simulink library "motohawk_control_primitives_lib"  (Simulink 7.5)
settings: Solver=ode45  SolverMode=SingleTasking  StartTime=0.0  StopTime=10.0  RelTol=1e-3
undefined symbols (not defined in the file): group, motohawk_vardec_config_group, motohawk_vardec_path, p, samp_time, SampleTime
libraries: MotoHawk_lib x103, motohawk_control_primitives_lib x29, simulink x11, AutoDoc_lib x4
(part 3 of 4)

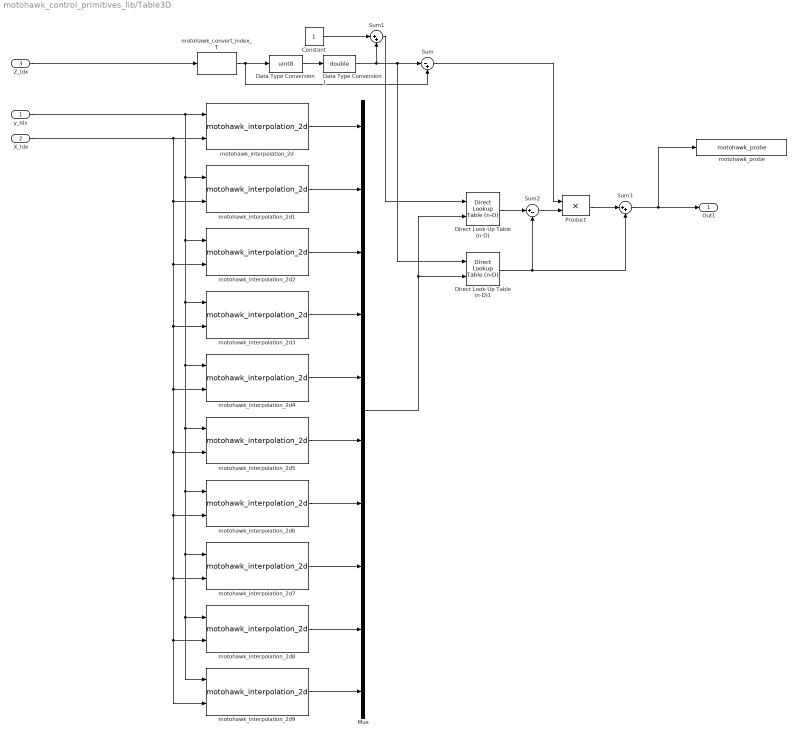
== system motohawk_control_primitives_lib/Table3D ==
  y_Idx : Inport  OutDataType=sfix(16)  OutScaling=2^0
  X_Idx : Inport  Port=2  OutDataType=sfix(16)  OutScaling=2^0
  Z_Idx : Inport  Port=3  OutDataType=sfix(16)  OutScaling=2^0
  Constant : Constant  OutDataType=sfix(16)  OutScaling=2^0
  Data Type Conversion : DataTypeConversion  OutDataTypeMode=uint8  OutDataType=sfix(16)  OutScaling=2^0  OutDataTypeStr=uint8  SaturateOnIntegerOverflow=on  RndMeth=Zero
  Data Type Conversion1 : DataTypeConversion  OutDataTypeMode=double  OutDataType=sfix(16)  OutScaling=2^0  OutDataTypeStr=double  SaturateOnIntegerOverflow=on  RndMeth=Zero
  Direct Look-Up Table (n-D) : simulink/Lookup Tables/Direct Lookup Table (n-D)  maskTabDims=1  explicitNumDims=1  outDims=Element  tabIsInput=on  mxTable=[4 5 6;16 19 20;10 18 23]  clipFlag=Warning
  Direct Look-Up Table (n-D)1 : simulink/Lookup Tables/Direct Lookup Table (n-D)  maskTabDims=1  explicitNumDims=1  outDims=Element  tabIsInput=on  mxTable=[4 5 6;16 19 20;10 18 23]  clipFlag=Warning
  Mux : Mux  Inputs=10
  Product : Product  OutDataType=sfix(16)  OutScaling=2^0  SaturateOnIntegerOverflow=on  OutDataTypeStr=Inherit: Same as first input
  Sum : Sum  Inputs=|-+  OutDataType=sfix(16)  OutScaling=2^0  SaturateOnIntegerOverflow=on
  Sum1 : Sum  Inputs=|++  OutDataType=sfix(16)  OutScaling=2^0  SaturateOnIntegerOverflow=on
  Sum2 : Sum  Inputs=|+-  OutDataType=sfix(16)  OutScaling=2^0  SaturateOnIntegerOverflow=on
  Sum3 : Sum  Inputs=|++  OutDataType=sfix(16)  OutScaling=2^0  SaturateOnIntegerOverflow=on
  motohawk_convert_index_T : MotoHawk_lib/Lookup Tables/motohawk_convert_index_T
  motohawk_interpolation_2d : MotoHawk_lib/Lookup Tables/motohawk_interpolation_2d  nam=[nam 'Z1']  table_data=table1data  show_more=on  data_type=Inherit from 'Table Data'  storage=NonAdaptive  read_level=1  write_level=1  ovr_cals=on  use_help=off  help=''  units=''  use_min_max=off  min_val=-inf  max_val=inf  use_precision=off  precision=''  gain=1  offset=0  exp=1  use_links=on  row_prelookup_block=rowprelookup  col_prelookup_block=colprelookup  output_name=''  use_mototune_group=on  mototune_group=grp
  motohawk_interpolation_2d1 : MotoHawk_lib/Lookup Tables/motohawk_interpolation_2d  nam=[nam 'Z2']  table_data=table2data  show_more=on  data_type=Inherit from 'Table Data'  storage=NonAdaptive  read_level=1  write_level=1  ovr_cals=on  use_help=off  help=''  units=''  use_min_max=off  min_val=-inf  max_val=inf  use_precision=off  precision=''  gain=1  offset=0  exp=1  use_links=on  row_prelookup_block=rowprelookup  col_prelookup_block=colprelookup  output_name=''  use_mototune_group=on  mototune_group=grp
  motohawk_interpolation_2d2 : MotoHawk_lib/Lookup Tables/motohawk_interpolation_2d  nam=[nam 'Z3']  table_data=table3data  show_more=on  data_type=Inherit from 'Table Data'  storage=NonAdaptive  read_level=1  write_level=1  ovr_cals=on  use_help=off  help=''  units=''  use_min_max=off  min_val=-inf  max_val=inf  use_precision=off  precision=''  gain=1  offset=0  exp=1  use_links=on  row_prelookup_block=rowprelookup  col_prelookup_block=colprelookup  output_name=''  use_mototune_group=on  mototune_group=grp
  motohawk_interpolation_2d3 : MotoHawk_lib/Lookup Tables/motohawk_interpolation_2d  nam=[nam 'Z4']  table_data=table4data  show_more=on  data_type=Inherit from 'Table Data'  storage=NonAdaptive  read_level=1  write_level=1  ovr_cals=on  use_help=off  help=''  units=''  use_min_max=off  min_val=-inf  max_val=inf  use_precision=off  precision=''  gain=1  offset=0  exp=1  use_links=on  row_prelookup_block=rowprelookup  col_prelookup_block=colprelookup  output_name=''  use_mototune_group=on  mototune_group=grp
  motohawk_interpolation_2d4 : MotoHawk_lib/Lookup Tables/motohawk_interpolation_2d  nam=[nam 'Z5']  table_data=table5data  show_more=on  data_type=Inherit from 'Table Data'  storage=NonAdaptive  read_level=1  write_level=1  ovr_cals=on  use_help=off  help=''  units=''  use_min_max=off  min_val=-inf  max_val=inf  use_precision=off  precision=''  gain=1  offset=0  exp=1  use_links=on  row_prelookup_block=rowprelookup  col_prelookup_block=colprelookup  output_name=''  use_mototune_group=on  mototune_group=grp
  motohawk_interpolation_2d5 : MotoHawk_lib/Lookup Tables/motohawk_interpolation_2d  nam=[nam 'Z6']  table_data=(table6data)  show_more=on  data_type=Inherit from 'Table Data'  storage=NonAdaptive  read_level=1  write_level=1  ovr_cals=on  use_help=off  help=''  units=''  use_min_max=off  min_val=-inf  max_val=inf  use_precision=off  precision=''  gain=1  offset=0  exp=1  use_links=on  row_prelookup_block=rowprelookup  col_prelookup_block=colprelookup  output_name=''  use_mototune_group=on  mototune_group=grp
  motohawk_interpolation_2d6 : MotoHawk_lib/Lookup Tables/motohawk_interpolation_2d  nam=[nam 'Z7']  table_data=(table7data)  show_more=on  data_type=Inherit from 'Table Data'  storage=NonAdaptive  read_level=1  write_level=1  ovr_cals=on  use_help=off  help=''  units=''  use_min_max=off  min_val=-inf  max_val=inf  use_precision=off  precision=''  gain=1  offset=0  exp=1  use_links=on  row_prelookup_block=rowprelookup  col_prelookup_block=colprelookup  output_name=''  use_mototune_group=on  mototune_group=grp
  motohawk_interpolation_2d7 : MotoHawk_lib/Lookup Tables/motohawk_interpolation_2d  nam=[nam 'Z8']  table_data=(table8data)  show_more=on  data_type=Inherit from 'Table Data'  storage=NonAdaptive  read_level=1  write_level=1  ovr_cals=on  use_help=off  help=''  units=''  use_min_max=off  min_val=-inf  max_val=inf  use_precision=off  precision=''  gain=1  offset=0  exp=1  use_links=on  row_prelookup_block=rowprelookup  col_prelookup_block=colprelookup  output_name=''  use_mototune_group=on  mototune_group=grp
  motohawk_interpolation_2d8 : MotoHawk_lib/Lookup Tables/motohawk_interpolation_2d  nam=[nam 'Z9']  table_data=(table9data)  show_more=on  data_type=Inherit from 'Table Data'  storage=NonAdaptive  read_level=1  write_level=1  ovr_cals=on  use_help=off  help=''  units=''  use_min_max=off  min_val=-inf  max_val=inf  use_precision=off  precision=''  gain=1  offset=0  exp=1  use_links=on  row_prelookup_block=rowprelookup  col_prelookup_block=colprelookup  output_name=''  use_mototune_group=on  mototune_group=grp
  motohawk_interpolation_2d9 : MotoHawk_lib/Lookup Tables/motohawk_interpolation_2d  nam=[nam 'Z10']  table_data=(table10data)  show_more=on  data_type=Inherit from 'Table Data'  storage=NonAdaptive  read_level=1  write_level=1  ovr_cals=on  use_help=off  help=''  units=''  use_min_max=off  min_val=-inf  max_val=inf  use_precision=off  precision=''  gain=1  offset=0  exp=1  use_links=on  row_prelookup_block=rowprelookup  col_prelookup_block=colprelookup  output_name=''  use_mototune_group=on  mototune_group=grp
  motohawk_probe : MotoHawk_lib/Calibration & Probing Blocks/motohawk_probe  nam=[nam]  show_more=on  name_source=Use Parameter  read_level=1  view_as=Number  enum_struct={'Disabled', 'Enabled'}  vector_style=Wide Row  use_help_units=off  help=''  units=''  use_header_enum=off  row_header_enum={}  col_header_enum={}  use_precision=off  precision=''  gain=1  offset=0  exp=1  use_mototune_group=on  mototune_group=grp
  Out1 : Outport  OutDataType=sfix(16)  OutScaling=2^0
  wires:
  Sum3/1 -> Out1/1, motohawk_probe/1
  Product/1 -> Sum3/1
  Direct Look-Up Table (n-D)1/1 -> Sum3/2, Sum2/2
  Direct Look-Up Table (n-D)/1 -> Sum2/1
  Sum1/1 -> Direct Look-Up Table (n-D)/1
  Constant/1 -> Sum1/1
  Data Type Conversion1/1 -> Direct Look-Up Table (n-D)1/1, Sum/1, Sum1/2
  Data Type Conversion/1 -> Data Type Conversion1/1
  motohawk_convert_index_T/1 -> Sum/2, Data Type Conversion/1
  motohawk_interpolation_2d3/1 -> Mux/4
  motohawk_interpolation_2d2/1 -> Mux/3
  motohawk_interpolation_2d1/1 -> Mux/2
  motohawk_interpolation_2d/1 -> Mux/1
  Z_Idx/1 -> motohawk_convert_index_T/1
  X_Idx/1 -> motohawk_interpolation_2d2/2, motohawk_interpolation_2d3/2, motohawk_interpolation_2d4/2, motohawk_interpolation_2d5/2, motohawk_interpolation_2d6/2, motohawk_interpolation_2d7/2, motohawk_interpolation_2d8/2, motohawk_interpolation_2d9/2, motohawk_interpolation_2d1/2, motohawk_interpolation_2d/2
  y_Idx/1 -> motohawk_interpolation_2d2/1, motohawk_interpolation_2d3/1, motohawk_interpolation_2d4/1, motohawk_interpolation_2d5/1, motohawk_interpolation_2d6/1, motohawk_interpolation_2d7/1, motohawk_interpolation_2d8/1, motohawk_interpolation_2d9/1, motohawk_interpolation_2d1/1, motohawk_interpolation_2d/1
  motohawk_interpolation_2d4/1 -> Mux/5
  motohawk_interpolation_2d5/1 -> Mux/6
  Sum/1 -> Product/1
  Sum2/1 -> Product/2
  motohawk_interpolation_2d6/1 -> Mux/7
  motohawk_interpolation_2d7/1 -> Mux/8
  motohawk_interpolation_2d8/1 -> Mux/9
  motohawk_interpolation_2d9/1 -> Mux/10
  Mux/1 -> Direct Look-Up Table (n-D)/2, Direct Look-Up Table (n-D)1/2

== system motohawk_control_primitives_lib/Time Since Enabled ==
  note: Output the time since enabled, by summing up 'dt'.
  note: If this block is in an enabled subsystem that
      | resets its states, then the count will reset as well.
      | Otherwise, the count will resume from where it left off.
      |
      | Note that when the Sample Time of the the 'dt' is non-positive,
      | the block will only output its Initial Value if the enabled subsystem
      | is set to reset its state.  This means that the count will immediately
      | 'catch up' if the enabled subsystem holds its states.
  Sum : Sum  Inputs=|++  OutDataType=sfix(16)  OutScaling=2^0  SaturateOnIntegerOverflow=on  InputSameDT=on
  Unit Delay : UnitDelay  SampleTime=-1
  motohawk_delta_time : MotoHawk_lib/Extra Development Blocks/motohawk_delta_time  samp_time=samp_time  init_val=0
  Time Since Enabled [sec] : Outport  OutDataType=sfix(16)  OutScaling=2^0
  wires:
  Unit Delay/1 -> Time Since Enabled [sec]/1, Sum/2
  Sum/1 -> Unit Delay/1
  motohawk_delta_time/1 -> Sum/1

== system motohawk_control_primitives_lib/Time Since Enabled (With Input) ==
  note: Output the time since enabled, by summing up 'dt'.
      | States are reset when re-enabled.
      | Output is reset to zero when disabled.
  Enable : EnablePort  StatesWhenEnabling=reset  ZeroCross=off
  Sum : Sum  Inputs=|++  OutDataType=sfix(16)  OutScaling=2^0  SaturateOnIntegerOverflow=on  InputSameDT=on
  Unit Delay : UnitDelay  SampleTime=-1
  motohawk_delta_time : MotoHawk_lib/Extra Development Blocks/motohawk_delta_time  samp_time=samp_time  init_val=0
  Time Since Enabled [sec] : Outport  OutDataType=sfix(16)  OutScaling=2^0  OutputWhenDisabled=reset  InitialOutput=init
  wires:
  motohawk_delta_time/1 -> Sum/1
  Sum/1 -> Unit Delay/1
  Unit Delay/1 -> Sum/2, Time Since Enabled [sec]/1

== system motohawk_control_primitives_lib/Time Since Enabled (With Input)1 ==
  Enable : Inport  OutDataType=sfix(16)  OutScaling=2^0
  Constant : Constant  Value=init  OutDataType=sfix(16)  OutScaling=2^0
  Saturation : Saturate  UpperLimit=upperlim  LowerLimit=0
  Sum : Sum  Inputs=++|  OutDataType=sfix(16)  OutScaling=2^0  SaturateOnIntegerOverflow=on  InputSameDT=on
  Switch : Switch  Threshold=1
  motohawk_data_def : MotoHawk_lib/Data Storage Blocks/motohawk_data_def  nam=nam  data=0  typ=double  struct_nam='MyStruct'  storage=Volatile  outputRef=off  use_vardec=off  window=Calibration  read_level=1  write_level=1  ovr_cals=on  view_as=Number  enum_struct={'Disabled', 'Enabled'}  vector_style=Wide Row  use_help_units=on  help=''  units=''  use_header_enum=off  row_header_enum=''  col_header_enum=''  use_min_max=off  min_val=-inf  max_val=inf  use_precision=off  precision=''  gain=1  offset=0  exp=1  use_mototune_group=off  mototune_group=motohawk_vardec_path(gcb)  eval_name=TimeSinceRun
  motohawk_data_read : MotoHawk_lib/Data Storage Blocks/motohawk_data_read  source=Lookup By Name  structure=Scalar  operation=Read scalar from location by index  sz_vec=4  sz_row=2  sz_col=3  typ=double  nam=nam  checkNull=on  struct_inst_name='Struct1'
  motohawk_data_write : MotoHawk_lib/Data Storage Blocks/motohawk_data_write  source=Lookup By Name  structure=Scalar  operation=Write scalar into location by index  sz_vec=-1  sz_row=3  sz_col=2  typ=double  nam=nam  checkNull=on  write_read_only=off  struct_inst_name='Struct1'
  motohawk_delta_time : MotoHawk_lib/Extra Development Blocks/motohawk_delta_time  samp_time=samp_time  init_val=.005
  Time : Outport  OutDataType=sfix(16)  OutScaling=2^0  OutputWhenDisabled=reset  InitialOutput=init
  wires:
  motohawk_delta_time/1 -> Sum/1
  motohawk_data_read/1 -> Sum/2
  Switch/1 -> Time/1, Saturation/1
  Enable/1 -> Switch/2
  Sum/1 -> Switch/1
  Constant/1 -> Switch/3
  Saturation/1 -> motohawk_data_write/1

== system motohawk_control_primitives_lib/Triggered Counter Falling ==
  note: Triggered Counter
  Reset : Inport  OutDataType=sfix(16)  OutScaling=2^0
  Increment : Inport  Port=2  OutDataType=sfix(16)  OutScaling=2^0
  Trigger : TriggerPort  TriggerType=falling
  Constant : Constant  Value=0  OutDataType=sfix(16)  OutScaling=2^0
  Sum : Sum  OutDataType=sfix(16)  OutScaling=2^0  SaturateOnIntegerOverflow=on  InputSameDT=on  OutDataTypeStr=Inherit: Same as first input
  Switch : Switch  Threshold=0.5  SaturateOnIntegerOverflow=on  InputSameDT=on
  Unit Delay1 : UnitDelay  SampleTime=-1
  Counter : Outport  OutDataType=sfix(16)  OutScaling=2^0
  wires:
  Unit Delay1/1 -> Sum/2
  Increment/1 -> Sum/1
  Reset/1 -> Switch/2
  Switch/1 -> Unit Delay1/1, Counter/1
  Constant/1 -> Switch/1
  Sum/1 -> Switch/3

== system motohawk_control_primitives_lib/Triggered Counter Rising ==
  note: Triggered Counter
  Reset : Inport  OutDataType=sfix(16)  OutScaling=2^0
  Increment : Inport  Port=2  OutDataType=sfix(16)  OutScaling=2^0
  Trigger : TriggerPort
  Constant : Constant  Value=0  OutDataType=sfix(16)  OutScaling=2^0
  Sum : Sum  OutDataType=sfix(16)  OutScaling=2^0  SaturateOnIntegerOverflow=on  InputSameDT=on  OutDataTypeStr=Inherit: Same as first input
  Switch : Switch  Threshold=0.5  SaturateOnIntegerOverflow=on  InputSameDT=on
  Unit Delay1 : UnitDelay  SampleTime=-1
  Counter : Outport  OutDataType=sfix(16)  OutScaling=2^0
  wires:
  Switch/1 -> Counter/1, Unit Delay1/1
  Reset/1 -> Switch/2
  Constant/1 -> Switch/1
  Sum/1 -> Switch/3
  Increment/1 -> Sum/1
  Unit Delay1/1 -> Sum/2

== system motohawk_control_primitives_lib/Universal PD ==
  note: Universal PD Controller
  Actual : Inport  OutDataType=sfix(16)  OutScaling=2^0
  SetPt : Inport  Port=2  OutDataType=sfix(16)  OutScaling=2^0
  k_Err : Inport  Port=3  OutDataType=sfix(16)  OutScaling=2^0
  k_P : Inport  Port=4  OutDataType=sfix(16)  OutScaling=2^0
  k_D : Inport  Port=5  OutDataType=sfix(16)  OutScaling=2^0
  Data Type Conversion : DataTypeConversion  OutDataType=sfix(16)  OutScaling=2^0  SaturateOnIntegerOverflow=on  RndMeth=Zero
  Derivitive : motohawk_control_primitives_lib/Derivitive  samp_time=samp_time
  Model Info : simulink/Model-Wide Utilities/Model Info  InitialBlockCM=None  BlockCM=None  Frame=on  DisplayStringWithTags=|  HorizontalTextAlignment=Center  LeftAlignmentValue=0.5  SourceBlockDiagram=motohawk_control_primitives_lib  TagMaxNumber=20
      | Model Info:
      | Author: %<Creator>
      | %<Created>
      | %<ModifiedDate>
      | Version: %<ModelVersion>
      | MotoTron Confidential
      | and Propietary
  Product : Product  OutDataType=sfix(16)  OutScaling=2^0  InputSameDT=on  OutDataTypeStr=Inherit: Same as first input
  Product2 : Product  OutDataType=sfix(16)  OutScaling=2^0  InputSameDT=on  OutDataTypeStr=Inherit: Same as first input
  Product4 : Product  OutDataType=sfix(16)  OutScaling=2^0  InputSameDT=on  OutDataTypeStr=Inherit: Same as first input
  Sum : Sum  OutDataType=sfix(16)  OutScaling=2^0  SaturateOnIntegerOverflow=on  InputSameDT=on  OutDataTypeStr=Inherit: Same as first input
  Sum1 : Sum  Inputs=|-+  OutDataType=sfix(16)  OutScaling=2^0
  Out : Outport  OutDataType=sfix(16)  OutScaling=2^0
  Err : Outport  Port=2  OutDataType=sfix(16)  OutScaling=2^0
  P_term : Outport  Port=3  OutDataType=sfix(16)  OutScaling=2^0
  D_term : Outport  Port=4  OutDataType=sfix(16)  OutScaling=2^0
  wires:
  Product4/1 -> Product2/1, Product/1
  Sum/1 -> Out/1
  Derivitive/1 -> Sum/2, D_term/1
  Product/1 -> Sum/1, P_term/1
  Product2/1 -> Derivitive/1
  k_D/1 -> Product2/2
  k_P/1 -> Product/2
  Actual/1 -> Sum1/1
  SetPt/1 -> Sum1/2
  Sum1/1 -> Data Type Conversion/1
  k_Err/1 -> Product4/2
  Data Type Conversion/1 -> Product4/1, Err/1

== system motohawk_control_primitives_lib/Universal PD (Tunable & Scheduled) ==
  note: Universal PD Feedback Control
      | With Calibratable Parameters,
      | Gain Schedules, and Observable States
  Actual : Inport  OutDataType=sfix(16)  OutScaling=2^0
  SetPoint : Inport  Port=2  OutDataType=sfix(16)  OutScaling=2^0
  Product1 : Product  OutDataType=sfix(16)  OutScaling=2^0  SaturateOnIntegerOverflow=on  InputSameDT=on  OutDataTypeStr=Inherit: Same as first input
  Product2 : Product  OutDataType=sfix(16)  OutScaling=2^0  SaturateOnIntegerOverflow=on  InputSameDT=on  OutDataTypeStr=Inherit: Same as first input
  Saturation (Tunable) : motohawk_control_primitives_lib/Saturation (Tunable)  prefix=prefix  units=units  grp=motohawk_vardec_config_group(grp)
  Sum : Sum  Inputs=++|  OutDataType=sfix(16)  OutScaling=2^0  InputSameDT=on
  Universal PD : motohawk_control_primitives_lib/Universal PD  Description=|  samp_time=SampleTime
      | /* Name: ErrorGain Unit:mult ClassID:VAR StorageID:FLASH Access:RW4+RW3+NA2+NA1 TypeID:UINT4                   
      |    Gain:0.000000001 Min:0.000000000 Max:4.000000000 Format:10.9 UpdateID:REMOTE Help:"This gain is applied to "
      |    "the error term before it is used to calculate the P, I and D terms." VardecSig:6C */                       
      |                                                                                                                
      | /* Name: ITermLowerLim Unit:0 ClassID:VAR StorageID:FLASH Access:RW4+RW3+NA2+NA1 TypeID:SINT2 Gain:0.1         
      |    Min:-3276.8 Max:3276.7 Format:5.1 UpdateID:REMOTE Help:"Lower limit on the I-term value." VardecSig:6C */   
      |                                                                                                                
      | /* Name: ITermUpperLim ClassID:VAR StorageID:FLASH Access:RW4+RW3+NA2+NA1 TypeID:SINT2 Gain:0.1 Min:-3276.8    
      |    Max:3276.7 Format:5.1 UpdateID:REMOTE Help:"Upper limit on I-term value." VardecSig:6C */                   
      |                                                                                                                
      | /* Name: PIDOutLowerLim ClassID:VAR StorageID:FLASH Access:RW4+RW3+NA2+NA1 TypeID:SINT2 Gain:0.1               
      |    Min:-3276.8 Max:3276.7 Format:5.1 UpdateID:REMOTE Help:"Lower limit on PID output." VardecSig:6C */         
      |                                                                                                                
      | /* Name: PIDOutUpperLim ClassID:VAR StorageID:FLASH Access:RW4+RW3+NA2+NA1 TypeID:SINT2 Gain:0.1               
      |    Min:-3276.8 Max:3276.7 Format:3.1 UpdateID:REMOTE Help:"Upper limit on PID output." VardecSig:6C */
  motohawk_calibration : MotoHawk_lib/Calibration & Probing Blocks/motohawk_calibration  nam=[prefix 'PGain']  val=1  storage=Calibration  show_more=on  name_source=Use Parameter  data_type=Inherit from 'Default Value'  read_level=1  write_level=1  ovr_cals=on  view_as=Number  enum_struct={'Disabled', 'Enabled'}  vector_style=Wide Row  use_help_units=on  help='PID Proportional Gain'  units='mult'  use_header_enum=off  row_header_enum={}  col_header_enum={}  use_min_max=off  min_val=-inf  max_val=inf  use_precision=off  precision=''  gain=1  offset=0  exp=1  use_mototune_group=on  mototune_group=motohawk_vardec_config_group(grp)
  motohawk_calibration1 : MotoHawk_lib/Calibration & Probing Blocks/motohawk_calibration  nam=[prefix 'DGain']  val=1  storage=Calibration  show_more=on  name_source=Use Parameter  data_type=Inherit from 'Default Value'  read_level=1  write_level=1  ovr_cals=on  view_as=Number  enum_struct={'Disabled', 'Enabled'}  vector_style=Wide Row  use_help_units=on  help='PID Derivative Gain'  units='mult'  use_header_enum=off  row_header_enum={}  col_header_enum={}  use_min_max=off  min_val=-inf  max_val=inf  use_precision=off  precision=''  gain=1  offset=0  exp=1  use_mototune_group=on  mototune_group=motohawk_vardec_config_group(grp)
  motohawk_calibration5 : MotoHawk_lib/Calibration & Probing Blocks/motohawk_calibration  nam=[prefix 'DCOffset']  val=0  storage=Calibration  show_more=on  name_source=Use Parameter  data_type=Inherit from 'Default Value'  read_level=1  write_level=1  ovr_cals=on  view_as=Number  enum_struct={'Disabled', 'Enabled'}  vector_style=Wide Row  use_help_units=on  help='PID Output DC Offset'  units=units  use_header_enum=off  row_header_enum={}  col_header_enum={}  use_min_max=off  min_val=-inf  max_val=inf  use_precision=off  precision=''  gain=1  offset=0  exp=1  use_mototune_group=on  mototune_group=motohawk_vardec_config_group(grp)
  motohawk_calibration6 : MotoHawk_lib/Calibration & Probing Blocks/motohawk_calibration  nam=[prefix 'ErrorGain']  val=1  storage=Calibration  show_more=on  name_source=Use Parameter  data_type=Inherit from 'Default Value'  read_level=1  write_level=1  ovr_cals=on  view_as=Number  enum_struct={'Disabled', 'Enabled'}  vector_style=Wide Row  use_help_units=on  help='PID Error Gain'  units='mult'  use_header_enum=off  row_header_enum={}  col_header_enum={}  use_min_max=off  min_val=-inf  max_val=inf  use_precision=off  precision=''  gain=1  offset=0  exp=1  use_mototune_group=on  mototune_group=motohawk_vardec_config_group(grp)
  motohawk_interpolation_1d : MotoHawk_lib/Lookup Tables/motohawk_interpolation_1d  nam=[prefix 'PMult']  table_data=ones(1,tblsize)  show_more=on  data_type=Inherit from 'Table Data'  storage=NonAdaptive  read_level=1  write_level=1  ovr_cals=on  use_help=on  help='Proportional term gain schedule'  units='mult'  use_min_max=off  min_val=-inf  max_val=inf  use_precision=off  precision=''  gain=1  offset=0  exp=1  use_links=off  prelookup_block=''  output_name=''  use_mototune_group=on  mototune_group=grp
  motohawk_interpolation_1d1 : MotoHawk_lib/Lookup Tables/motohawk_interpolation_1d  nam=[prefix 'DMult']  table_data=ones(1,tblsize)  show_more=on  data_type=Inherit from 'Table Data'  storage=NonAdaptive  read_level=1  write_level=1  ovr_cals=on  use_help=on  help='Derivative term gain schedule'  units='mult'  use_min_max=off  min_val=-inf  max_val=inf  use_precision=off  precision=''  gain=1  offset=0  exp=1  use_links=off  prelookup_block=''  output_name=''  use_mototune_group=on  mototune_group=grp
  motohawk_prelookup : MotoHawk_lib/Lookup Tables/motohawk_prelookup  nam=[prefix 'Error']  breakpoint_data=ones(1,tblsize)  show_more=on  data_type=Inherit from 'Table Data'  storage=Constant  read_level=1  write_level=1  ovr_cals=on  use_help=on  help='Error gain schedule ordinates'  units=units  use_min_max=off  min_val=-inf  max_val=inf  use_precision=off  precision=''  gain=1  offset=0  exp=1  use_links=on  input_name=[prefix 'Error']  use_mototune_group=on  mototune_group=grp
  motohawk_probe : MotoHawk_lib/Calibration & Probing Blocks/motohawk_probe  nam=[prefix 'Out']  show_more=on  name_source=Use Parameter  read_level=1  view_as=Number  enum_struct={'Disabled', 'Enabled'}  vector_style=Wide Row  use_help_units=on  help='PID Final Output'  units=units  use_header_enum=off  row_header_enum={}  col_header_enum={}  use_precision=off  precision=''  gain=1  offset=0  exp=1  use_mototune_group=on  mototune_group=grp
  motohawk_probe1 : MotoHawk_lib/Calibration & Probing Blocks/motohawk_probe  nam=[prefix 'PTerm']  show_more=on  name_source=Use Parameter  read_level=1  view_as=Number  enum_struct={'Disabled', 'Enabled'}  vector_style=Wide Row  use_help_units=on  help='PID Proportional Term'  units=units  use_header_enum=off  row_header_enum={}  col_header_enum={}  use_precision=off  precision=''  gain=1  offset=0  exp=1  use_mototune_group=on  mototune_group=grp
  motohawk_probe3 : MotoHawk_lib/Calibration & Probing Blocks/motohawk_probe  nam=[prefix 'DTerm']  show_more=on  name_source=Use Parameter  read_level=1  view_as=Number  enum_struct={'Disabled', 'Enabled'}  vector_style=Wide Row  use_help_units=on  help='PID Derivative Term'  units=units  use_header_enum=off  row_header_enum={}  col_header_enum={}  use_precision=off  precision=''  gain=1  offset=0  exp=1  use_mototune_group=on  mototune_group=grp
  motohawk_probe4 : MotoHawk_lib/Calibration & Probing Blocks/motohawk_probe  nam=[prefix 'Error']  show_more=on  name_source=Use Parameter  read_level=1  view_as=Number  enum_struct={'Disabled', 'Enabled'}  vector_style=Wide Row  use_help_units=on  help='PID Error Term'  units=units  use_header_enum=off  row_header_enum={}  col_header_enum={}  use_precision=off  precision=''  gain=1  offset=0  exp=1  use_mototune_group=on  mototune_group=grp
  Out : Outport  OutDataType=sfix(16)  OutScaling=2^0
  wires:
  motohawk_prelookup/1 -> motohawk_interpolation_1d1/1, motohawk_interpolation_1d/1
  SetPoint/1 -> Universal PD/2
  Actual/1 -> Universal PD/1
  Saturation (Tunable)/1 -> motohawk_probe/1, Out/1
  Universal PD/2 -> motohawk_prelookup/1, motohawk_probe4/1
  Universal PD/4 -> motohawk_probe3/1
  Universal PD/1 -> Sum/2
  Universal PD/3 -> motohawk_probe1/1
  Sum/1 -> Saturation (Tunable)/1
  motohawk_calibration5/1 -> Sum/1
  motohawk_calibration6/1 -> Universal PD/3
  Product2/1 -> Universal PD/4
  motohawk_calibration/1 -> Product2/1
  Product1/1 -> Universal PD/5
  motohawk_calibration1/1 -> Product1/1
  motohawk_interpolation_1d/1 -> Product2/2
  motohawk_interpolation_1d1/1 -> Product1/2

== system motohawk_control_primitives_lib/Universal PD (Tunable) ==
  note: Universal PD Feedback Control
      | With Calibratable Parameters and Observable States
  Actual : Inport  OutDataType=sfix(16)  OutScaling=2^0
  SetPoint : Inport  Port=2  OutDataType=sfix(16)  OutScaling=2^0
  Saturation (Tunable) : motohawk_control_primitives_lib/Saturation (Tunable)  prefix=prefix  units=units  grp=grp
  Sum : Sum  Inputs=++|  OutDataType=sfix(16)  OutScaling=2^0  InputSameDT=on
  Universal PD : motohawk_control_primitives_lib/Universal PD  Description=|  samp_time=SampleTime
      | /* Name: ErrorGain Unit:mult ClassID:VAR StorageID:FLASH Access:RW4+RW3+NA2+NA1 TypeID:UINT4                   
      |    Gain:0.000000001 Min:0.000000000 Max:4.000000000 Format:10.9 UpdateID:REMOTE Help:"This gain is applied to "
      |    "the error term before it is used to calculate the P, I and D terms." VardecSig:6C */                       
      |                                                                                                                
      | /* Name: ITermLowerLim Unit:0 ClassID:VAR StorageID:FLASH Access:RW4+RW3+NA2+NA1 TypeID:SINT2 Gain:0.1         
      |    Min:-3276.8 Max:3276.7 Format:5.1 UpdateID:REMOTE Help:"Lower limit on the I-term value." VardecSig:6C */   
      |                                                                                                                
      | /* Name: ITermUpperLim ClassID:VAR StorageID:FLASH Access:RW4+RW3+NA2+NA1 TypeID:SINT2 Gain:0.1 Min:-3276.8    
      |    Max:3276.7 Format:5.1 UpdateID:REMOTE Help:"Upper limit on I-term value." VardecSig:6C */                   
      |                                                                                                                
      | /* Name: PIDOutLowerLim ClassID:VAR StorageID:FLASH Access:RW4+RW3+NA2+NA1 TypeID:SINT2 Gain:0.1               
      |    Min:-3276.8 Max:3276.7 Format:5.1 UpdateID:REMOTE Help:"Lower limit on PID output." VardecSig:6C */         
      |                                                                                                                
      | /* Name: PIDOutUpperLim ClassID:VAR StorageID:FLASH Access:RW4+RW3+NA2+NA1 TypeID:SINT2 Gain:0.1               
      |    Min:-3276.8 Max:3276.7 Format:3.1 UpdateID:REMOTE Help:"Upper limit on PID output." VardecSig:6C */
  motohawk_calibration : MotoHawk_lib/Calibration & Probing Blocks/motohawk_calibration  nam=[prefix 'PGain']  val=1  storage=Calibration  show_more=on  name_source=Use Parameter  data_type=Inherit from 'Default Value'  read_level=1  write_level=1  ovr_cals=on  view_as=Number  enum_struct={'Disabled', 'Enabled'}  vector_style=Wide Row  use_help_units=on  help='PID Proportional Gain'  units='mult'  use_header_enum=off  row_header_enum={}  col_header_enum={}  use_min_max=off  min_val=-inf  max_val=inf  use_precision=off  precision=''  gain=1  offset=0  exp=1  use_mototune_group=on  mototune_group=grp
  motohawk_calibration1 : MotoHawk_lib/Calibration & Probing Blocks/motohawk_calibration  nam=[prefix 'DGain']  val=1  storage=Calibration  show_more=on  name_source=Use Parameter  data_type=Inherit from 'Default Value'  read_level=1  write_level=1  ovr_cals=on  view_as=Number  enum_struct={'Disabled', 'Enabled'}  vector_style=Wide Row  use_help_units=on  help='PID Derivative Gain'  units='mult'  use_header_enum=off  row_header_enum={}  col_header_enum={}  use_min_max=off  min_val=-inf  max_val=inf  use_precision=off  precision=''  gain=1  offset=0  exp=1  use_mototune_group=on  mototune_group=grp
  motohawk_calibration5 : MotoHawk_lib/Calibration & Probing Blocks/motohawk_calibration  nam=[prefix 'DCOffset']  val=0  storage=Calibration  show_more=on  name_source=Use Parameter  data_type=Inherit from 'Default Value'  read_level=1  write_level=1  ovr_cals=on  view_as=Number  enum_struct={'Disabled', 'Enabled'}  vector_style=Wide Row  use_help_units=on  help='PID Output DC Offset'  units=units  use_header_enum=off  row_header_enum={}  col_header_enum={}  use_min_max=off  min_val=-inf  max_val=inf  use_precision=off  precision=''  gain=1  offset=0  exp=1  use_mototune_group=on  mototune_group=grp
  motohawk_calibration6 : MotoHawk_lib/Calibration & Probing Blocks/motohawk_calibration  nam=[prefix 'ErrorGain']  val=1  storage=Calibration  show_more=on  name_source=Use Parameter  data_type=Inherit from 'Default Value'  read_level=1  write_level=1  ovr_cals=on  view_as=Number  enum_struct={'Disabled', 'Enabled'}  vector_style=Wide Row  use_help_units=on  help='PID Error Gain'  units='mult'  use_header_enum=off  row_header_enum={}  col_header_enum={}  use_min_max=off  min_val=-inf  max_val=inf  use_precision=off  precision=''  gain=1  offset=0  exp=1  use_mototune_group=on  mototune_group=grp
  motohawk_probe : MotoHawk_lib/Calibration & Probing Blocks/motohawk_probe  nam=[prefix 'Out']  show_more=on  name_source=Use Parameter  read_level=1  view_as=Number  enum_struct={'Disabled', 'Enabled'}  vector_style=Wide Row  use_help_units=on  help='PID Final Output'  units=units  use_header_enum=off  row_header_enum={}  col_header_enum={}  use_precision=off  precision=''  gain=1  offset=0  exp=1  use_mototune_group=on  mototune_group=grp
  motohawk_probe1 : MotoHawk_lib/Calibration & Probing Blocks/motohawk_probe  nam=[prefix 'PTerm']  show_more=on  name_source=Use Parameter  read_level=1  view_as=Number  enum_struct={'Disabled', 'Enabled'}  vector_style=Wide Row  use_help_units=on  help='PID Proportional Term'  units=units  use_header_enum=off  row_header_enum={}  col_header_enum={}  use_precision=off  precision=''  gain=1  offset=0  exp=1  use_mototune_group=on  mototune_group=grp
  motohawk_probe3 : MotoHawk_lib/Calibration & Probing Blocks/motohawk_probe  nam=[prefix 'DTerm']  show_more=on  name_source=Use Parameter  read_level=1  view_as=Number  enum_struct={'Disabled', 'Enabled'}  vector_style=Wide Row  use_help_units=on  help='PID Derivative Term'  units=units  use_header_enum=off  row_header_enum={}  col_header_enum={}  use_precision=off  precision=''  gain=1  offset=0  exp=1  use_mototune_group=on  mototune_group=grp
  motohawk_probe4 : MotoHawk_lib/Calibration & Probing Blocks/motohawk_probe  nam=[prefix 'Error']  show_more=on  name_source=Use Parameter  read_level=1  view_as=Number  enum_struct={'Disabled', 'Enabled'}  vector_style=Wide Row  use_help_units=on  help='PID Error Term'  units=units  use_header_enum=off  row_header_enum={}  col_header_enum={}  use_precision=off  precision=''  gain=1  offset=0  exp=1  use_mototune_group=on  mototune_group=grp
  Out : Outport  OutDataType=sfix(16)  OutScaling=2^0
  wires:
  motohawk_calibration5/1 -> Sum/1
  Sum/1 -> Saturation (Tunable)/1
  Universal PD/3 -> motohawk_probe1/1
  Universal PD/1 -> Sum/2
  Universal PD/4 -> motohawk_probe3/1
  Universal PD/2 -> motohawk_probe4/1
  Saturation (Tunable)/1 -> Out/1, motohawk_probe/1
  motohawk_calibration6/1 -> Universal PD/3
  motohawk_calibration/1 -> Universal PD/4
  motohawk_calibration1/1 -> Universal PD/5
  Actual/1 -> Universal PD/1
  SetPoint/1 -> Universal PD/2

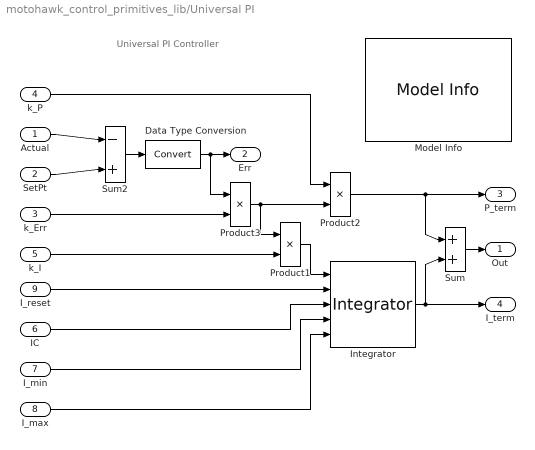
== system motohawk_control_primitives_lib/Universal PI ==
  note: Universal PI Controller
  Actual : Inport  OutDataType=sfix(16)  OutScaling=2^0
  SetPt : Inport  Port=2  OutDataType=sfix(16)  OutScaling=2^0
  k_Err : Inport  Port=3  OutDataType=sfix(16)  OutScaling=2^0
  k_P : Inport  Port=4  OutDataType=sfix(16)  OutScaling=2^0
  k_I : Inport  Port=5  OutDataType=sfix(16)  OutScaling=2^0
  IC : Inport  Port=6  OutDataType=sfix(16)  OutScaling=2^0
  I_min : Inport  Port=7  OutDataType=sfix(16)  OutScaling=2^0
  I_max : Inport  Port=8  OutDataType=sfix(16)  OutScaling=2^0
  I_reset : Inport  Port=9  OutDataType=sfix(16)  OutScaling=2^0
  Data Type Conversion : DataTypeConversion  OutDataType=sfix(16)  OutScaling=2^0  SaturateOnIntegerOverflow=on  RndMeth=Zero
  Integrator : motohawk_control_primitives_lib/Integrator  samp_time=samp_time
  Model Info : simulink/Model-Wide Utilities/Model Info  InitialBlockCM=None  BlockCM=None  Frame=on  DisplayStringWithTags=|  HorizontalTextAlignment=Center  LeftAlignmentValue=0.5  SourceBlockDiagram=motohawk_control_primitives_lib  TagMaxNumber=20
      | Model Info:
      | Author: Poorman
      | %<Created>
      | %<ModifiedDate>
      | Version: %<ModelVersion>
      | MotoTron Confidential
      | and Propietary
  Product1 : Product  OutDataType=sfix(16)  OutScaling=2^0  InputSameDT=on  OutDataTypeStr=Inherit: Same as first input
  Product2 : Product  OutDataType=sfix(16)  OutScaling=2^0  InputSameDT=on  OutDataTypeStr=Inherit: Same as first input
  Product3 : Product  OutDataType=sfix(16)  OutScaling=2^0  InputSameDT=on  OutDataTypeStr=Inherit: Same as first input
  Sum : Sum  Inputs=+|+  OutDataType=sfix(16)  OutScaling=2^0  SaturateOnIntegerOverflow=on  InputSameDT=on  OutDataTypeStr=Inherit: Same as first input
  Sum2 : Sum  Inputs=-|+  OutDataType=sfix(16)  OutScaling=2^0  SaturateOnIntegerOverflow=on  InputSameDT=on  OutDataTypeStr=Inherit: Same as first input
  Out : Outport  OutDataType=sfix(16)  OutScaling=2^0
  Err : Outport  Port=2  OutDataType=sfix(16)  OutScaling=2^0
  P_term : Outport  Port=3  OutDataType=sfix(16)  OutScaling=2^0
  I_term : Outport  Port=4  OutDataType=sfix(16)  OutScaling=2^0
  wires:
  I_max/1 -> Integrator/5
  I_min/1 -> Integrator/4
  Data Type Conversion/1 -> Err/1, Product3/1
  k_Err/1 -> Product3/2
  I_reset/1 -> Integrator/2
  SetPt/1 -> Sum2/2
  Actual/1 -> Sum2/1
  k_P/1 -> Product2/1
  k_I/1 -> Product1/2
  Product1/1 -> Integrator/1
  Product2/1 -> P_term/1, Sum/1
  Integrator/1 -> I_term/1, Sum/2
  Sum/1 -> Out/1
  IC/1 -> Integrator/3
  Product3/1 -> Product2/2, Product1/1
  Sum2/1 -> Data Type Conversion/1

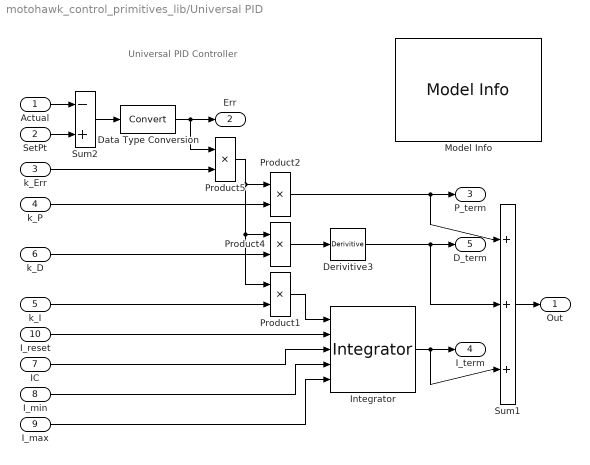
== system motohawk_control_primitives_lib/Universal PID ==
  note: Universal PID Controller
  Actual : Inport  OutDataType=sfix(16)  OutScaling=2^0
  SetPt : Inport  Port=2  OutDataType=sfix(16)  OutScaling=2^0
  k_Err : Inport  Port=3  OutDataType=sfix(16)  OutScaling=2^0
  k_P : Inport  Port=4  OutDataType=sfix(16)  OutScaling=2^0
  k_I : Inport  Port=5  OutDataType=sfix(16)  OutScaling=2^0
  k_D : Inport  Port=6  OutDataType=sfix(16)  OutScaling=2^0
  IC : Inport  Port=7  OutDataType=sfix(16)  OutScaling=2^0
  I_min : Inport  Port=8  OutDataType=sfix(16)  OutScaling=2^0
  I_max : Inport  Port=9  OutDataType=sfix(16)  OutScaling=2^0
  I_reset : Inport  Port=10  OutDataType=sfix(16)  OutScaling=2^0
  Data Type Conversion : DataTypeConversion  OutDataType=sfix(16)  OutScaling=2^0  SaturateOnIntegerOverflow=on  RndMeth=Zero
  Derivitive3 : motohawk_control_primitives_lib/Derivitive  samp_time=samp_time
  Integrator : motohawk_control_primitives_lib/Integrator  samp_time=samp_time
  Model Info : simulink/Model-Wide Utilities/Model Info  InitialBlockCM=None  BlockCM=None  Frame=on  DisplayStringWithTags=|  HorizontalTextAlignment=Center  LeftAlignmentValue=0.5  SourceBlockDiagram=motohawk_control_primitives_lib  TagMaxNumber=20
      | Model Info:
      | Author: Suhre, Poorman
      | %<Created>
      | %<ModifiedDate>
      | Version: %<ModelVersion>
      | MotoTron Confidential
      | and Propietary
  Product{1..2,4..5} (4 alike) : Product  OutDataType=sfix(16)  OutScaling=2^0  InputSameDT=on  OutDataTypeStr=Inherit: Same as first input
  Sum1 : Sum  Inputs=+|+|+  OutDataType=sfix(16)  OutScaling=2^0  SaturateOnIntegerOverflow=on  InputSameDT=on  OutDataTypeStr=Inherit: Same as first input
  Sum2 : Sum  Inputs=-+  OutDataType=sfix(16)  OutScaling=2^0  SaturateOnIntegerOverflow=on  InputSameDT=on  OutDataTypeStr=Inherit: Same as first input
  Out : Outport  OutDataType=sfix(16)  OutScaling=2^0
  Err : Outport  Port=2  OutDataType=sfix(16)  OutScaling=2^0
  P_term : Outport  Port=3  OutDataType=sfix(16)  OutScaling=2^0
  I_term : Outport  Port=4  OutDataType=sfix(16)  OutScaling=2^0
  D_term : Outport  Port=5  OutDataType=sfix(16)  OutScaling=2^0
  wires:
  I_max/1 -> Integrator/5
  I_min/1 -> Integrator/4
  Data Type Conversion/1 -> Product5/1, Err/1
  k_Err/1 -> Product5/2
  I_reset/1 -> Integrator/2
  Actual/1 -> Sum2/1
  k_P/1 -> Product2/2
  k_I/1 -> Product1/2
  Product1/1 -> Integrator/1
  Product2/1 -> P_term/1, Sum1/1
  Sum1/1 -> Out/1
  IC/1 -> Integrator/3
  Product5/1 -> Product2/1, Product1/1, Product4/1
  Sum2/1 -> Data Type Conversion/1
  SetPt/1 -> Sum2/2
  Product4/1 -> Derivitive3/1
  Derivitive3/1 -> D_term/1, Sum1/2
  k_D/1 -> Product4/2
  Integrator/1 -> I_term/1, Sum1/3
